simulink model "LastModelb4gameday"  (R2022b)
settings: Solver=FixedStepAuto  StartTime=0.0  StopTime=inf  RelTol=1e-3  EnableMultiTasking=on
libraries: vexarmcortexlib x18
settings Model: ExtModeTrigDuration=25  Creator=Mihai Nicoara  LastModifiedBy=bobsi
settings SolverCC: AutoInsertRateTranBlk=on
settings OptimizationCC: EnhancedBackFolding=on  PassReuseOutputArgsAs=Individual arguments  ZeroExternalMemoryAtStartup=off  ZeroInternalMemoryAtStartup=off  MaxStackSize=64  OptimizeBlockOrder=speed  DifferentSizesBufferReuse=on  OptimizationCustomize=off  EfficientTunableParamExpr=on
settings DebuggingCC: ParameterTunabilityLossMsg=error
settings HardwareCC: ProdBitPerPointer=32  ProdBitPerSizeT=32  ProdBitPerPtrDiffT=32  ProdLargestAtomicInteger=Long  ProdLargestAtomicFloat=Double  ProdWordSize=32  ProdHWDeviceType=ARM Compatible->ARM Cortex
settings SFSimCC: MATLABDynamicMemAlloc=off
settings RTWCC: Description=Embedded Coder  SystemTargetFile=ert.tlc  HardwareBoard=ARM Cortex-based VEX Microcontroller  TLCOptions="-aInlineSetEventsForThisBaseRateFcn=TLC_FALSE -aSuppressMultiTaskScheduler=TLC_FALSE  -aRateBasedStepFcn=0"  TemplateMakefile=ert_default_tmf  Toolchain=GNU Tools for VEX ARM Cortex
settings CodeAppCC: ForceParamTrailComments=on  IgnoreCustomStorageClasses=off  OperatorAnnotations=on  SimulinkDataObjDesc=on  SFDataObjDesc=on  InsertBlockDesc=on
settings ERTTargetCC: ExtModeTransport=1  ExtModeMexFile=ext_serial_win32_comm

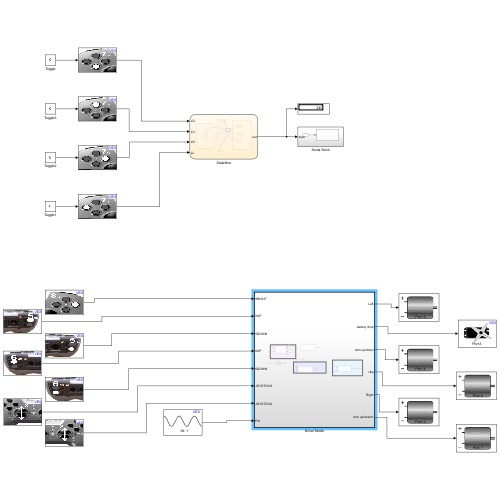
[thumbnail: Simulink's stored preview of the top-level diagram]
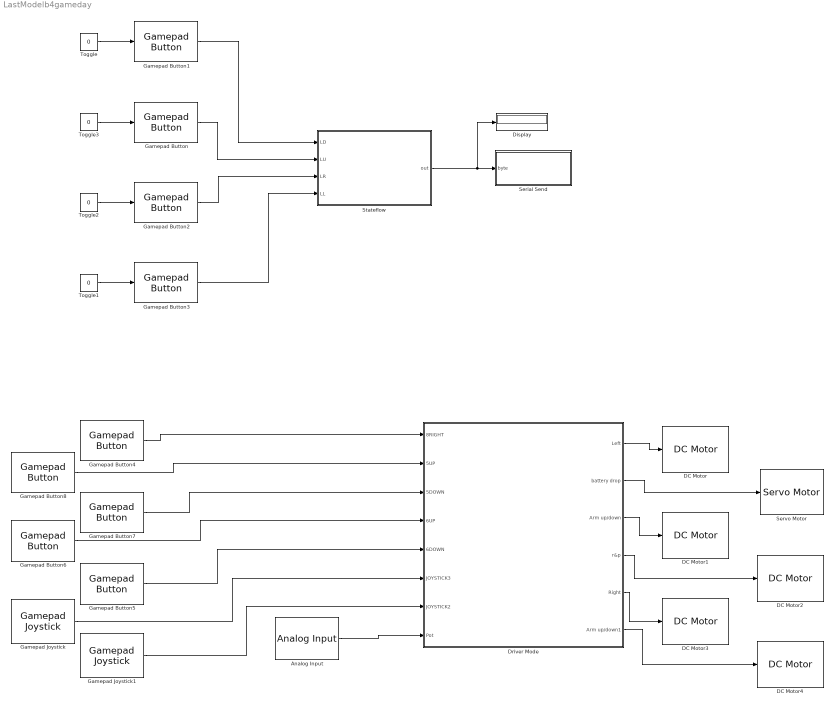
== system LastModelb4gameday ==
  Analog Input : vexarmcortexlib/Sensors/Analog Input  inChan=1  SimulationIn=off  SampleTime=0.02
  DC Motor : vexarmcortexlib/Actuators/DC Motor  motor=9  scaleFactor=1/13.5  SimulationOut=off
  DC Motor1 : vexarmcortexlib/Actuators/DC Motor  motor=4  scaleFactor=1/13.5  SimulationOut=off
  DC Motor2 : vexarmcortexlib/Actuators/DC Motor  motor=6  scaleFactor=1/13.5  SimulationOut=off
  DC Motor3 : vexarmcortexlib/Actuators/DC Motor  motor=2  scaleFactor=1/13.5  SimulationOut=off
  DC Motor4 : vexarmcortexlib/Actuators/DC Motor  motor=7  scaleFactor=1/13.5  SimulationOut=off
  Display : Display
  Driver Mode : Subsystem  TreatAsAtomicUnit=on
  Gamepad Button : vexarmcortexlib/Gamepad/Gamepad Button  joystick=1  chan=7  button56=Up  button78=Up  SimulationIn=on  SampleTime=0.02
  Gamepad Button1 : vexarmcortexlib/Gamepad/Gamepad Button  joystick=1  chan=7  button56=Up  button78=Down  SimulationIn=on  SampleTime=0.02
  Gamepad Button2 : vexarmcortexlib/Gamepad/Gamepad Button  joystick=1  chan=7  button56=Up  button78=Right  SimulationIn=on  SampleTime=0.02
  Gamepad Button3 : vexarmcortexlib/Gamepad/Gamepad Button  joystick=1  chan=7  button56=Up  button78=Left  SimulationIn=on  SampleTime=0.02
  Gamepad Button4 : vexarmcortexlib/Gamepad/Gamepad Button  joystick=1  chan=8  button56=Up  button78=Right  SimulationIn=off  SampleTime=0.02
  Gamepad Button5 : vexarmcortexlib/Gamepad/Gamepad Button  joystick=1  chan=6  button56=Down  button78=Left  SimulationIn=off  SampleTime=0.02
  Gamepad Button6 : vexarmcortexlib/Gamepad/Gamepad Button  joystick=1  chan=6  button56=Up  button78=Left  SimulationIn=off  SampleTime=0.02
  Gamepad Button7 : vexarmcortexlib/Gamepad/Gamepad Button  joystick=1  chan=5  button56=Down  button78=Left  SimulationIn=off  SampleTime=0.02
  Gamepad Button8 : vexarmcortexlib/Gamepad/Gamepad Button  joystick=1  chan=5  button56=Up  button78=Left  SimulationIn=off  SampleTime=0.02
  Gamepad Joystick : vexarmcortexlib/Gamepad/Gamepad Joystick  joystick=1  chan=3  SimulationIn=off  SampleTime=0.02
  Gamepad Joystick1 : vexarmcortexlib/Gamepad/Gamepad Joystick  joystick=1  chan=2  SimulationIn=off  SampleTime=0.02
  Serial Send : Subsystem
  Servo Motor : vexarmcortexlib/Actuators/Servo Motor  motor=3  scaleFactor=60/127  SimulationOut=off
  Stateflow : Stateflow chart  TreatAsAtomicUnit=on
  Toggle{,1..3} (4 alike) : Constant  Value=0
      settings: OpenFcn=|
      | if strcmp('0',get_param(gcb, 'Value'))                        set_param(gcb, 'Value', '1');
      | else
      |             set_param(gcb, 'Value', '0');
      | end
  wires:
  Gamepad Button/1 -> Stateflow/2(LU)
  Stateflow/1(out) -> Display/1, Serial Send/1(byte)
  Gamepad Button2/1 -> Stateflow/3(LR)
  Gamepad Button3/1 -> Stateflow/4(LL)
  Gamepad Button1/1 -> Stateflow/1(LD)
  Toggle/1 -> Gamepad Button1/1
  Toggle3/1 -> Gamepad Button/1
  Toggle2/1 -> Gamepad Button2/1
  Toggle1/1 -> Gamepad Button3/1
  Gamepad Button4/1 -> Driver Mode/1(8RIGHT)
  Gamepad Button8/1 -> Driver Mode/2(5UP)
  Gamepad Button7/1 -> Driver Mode/3(5DOWN)
  Gamepad Button6/1 -> Driver Mode/4(6UP)
  Gamepad Button5/1 -> Driver Mode/5(6DOWN)
  Gamepad Joystick/1 -> Driver Mode/6(JOYSTICK3)
  Gamepad Joystick1/1 -> Driver Mode/7(JOYSTICK2)
  Driver Mode/1(Left) -> DC Motor/1
  Driver Mode/5(Right) -> DC Motor3/1
  Driver Mode/3(Arm up/down) -> DC Motor1/1
  Driver Mode/2(battery drop) -> Servo Motor/1
  Driver Mode/4(r&p) -> DC Motor2/1
  Driver Mode/6(Arm up/down1) -> DC Motor4/1
  Analog Input/1 -> Driver Mode/8(Pot)

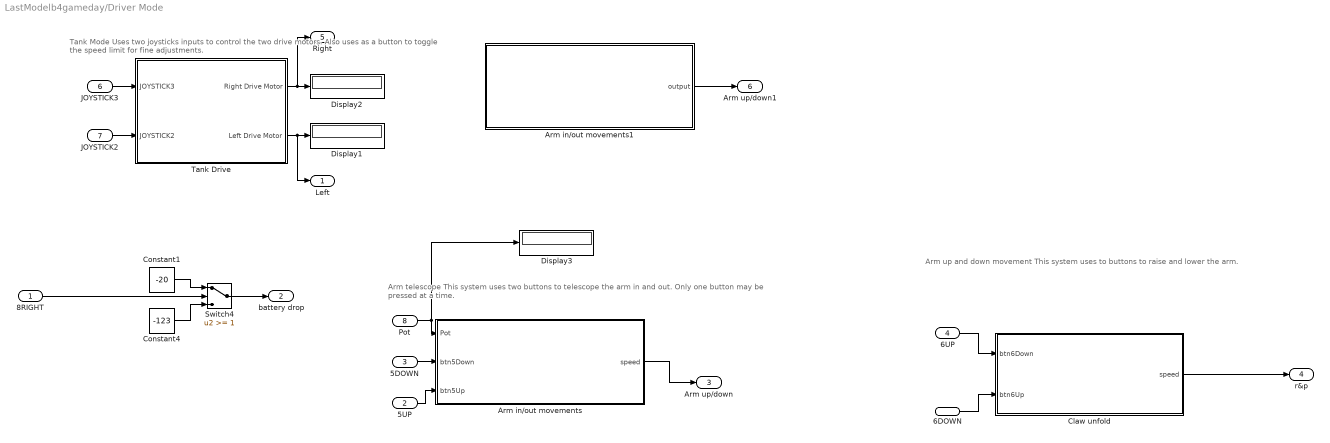
== system LastModelb4gameday/Driver Mode ==
  note: Tank Mode
      | Uses two joysticks inputs to control the two drive motors. Also uses as a button
      | to toggle the speed limit for fine adjustments.
  note: Arm up and down movement
      | This system uses to buttons to raise and lower the arm.
  note: Arm telescope
      | This system uses two buttons to telescope the arm in and out.
      | Only one button may be pressed at a time.
  8RIGHT : Inport
  5UP : Inport  Port=2
  5DOWN : Inport  Port=3
  6UP : Inport  Port=4
  6DOWN : Inport  Port=5
  JOYSTICK3 : Inport  Port=6
  JOYSTICK2 : Inport  Port=7
  Pot : Inport  Port=8
  Arm in/out movements : Stateflow chart  TreatAsAtomicUnit=on
  Arm in/out movements1 : Stateflow chart  TreatAsAtomicUnit=on
  Claw unfold : Stateflow chart  TreatAsAtomicUnit=on
  Constant1 : Constant  Value=-20
  Constant4 : Constant  Value=-123
  Display1 : Display
  Display2 : Display
  Display3 : Display
  Switch4 : Switch  Threshold=1  SaturateOnIntegerOverflow=off  InputSameDT=off
  "Tank Drive " : Subsystem  TreatAsAtomicUnit=on
  Left : Outport
  battery drop : Outport  Port=2
  Arm up/down : Outport  Port=3
  r&p : Outport  Port=4
  Right : Outport  Port=5
  Arm up/down1 : Outport  Port=6
  wires:
  Constant1/1 -> Switch4/1
  Claw unfold/1(speed) -> r&p/1
  Switch4/1 -> battery drop/1
  "Tank Drive "/2(Left Drive Motor) -> Left/1, Display1/1
  "Tank Drive "/1(Right Drive Motor) -> Right/1, Display2/1
  JOYSTICK2/1 -> "Tank Drive "/2(JOYSTICK2)
  8RIGHT/1 -> Switch4/2
  JOYSTICK3/1 -> "Tank Drive "/1(JOYSTICK3)
  Arm in/out movements/1(speed) -> Arm up/down/1
  Constant4/1 -> Switch4/3
  6UP/1 -> Claw unfold/1(btn6Down)
  6DOWN/1 -> Claw unfold/2(btn6Up)
  5UP/1 -> Arm in/out movements/3(btn5Up)
  5DOWN/1 -> Arm in/out movements/2(btn5Down)
  Pot/1 -> Arm in/out movements/1(Pot), Display3/1
  Arm in/out movements1/1(output) -> Arm up/down1/1

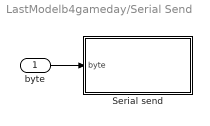
== system LastModelb4gameday/Serial Send ==
  byte : Inport  OutDataTypeStr=uint8  PortDimensions=[1 1]
  Serial send : MATLAB Function  TreatAsAtomicUnit=on
  wires:
  byte/1 -> Serial send/1(byte)

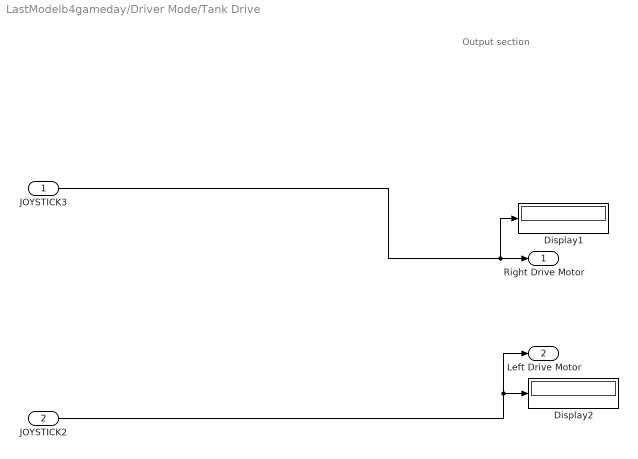
== system LastModelb4gameday/Driver Mode/Tank Drive  ==
  note: Output section
  JOYSTICK3 : Inport
  JOYSTICK2 : Inport  Port=2
  Display1 : Display
  Display2 : Display
  Right Drive Motor : Outport
  Left Drive Motor : Outport  Port=2
  wires:
  JOYSTICK3/1 -> Display1/1, Right Drive Motor/1
  JOYSTICK2/1 -> Display2/1, Left Drive Motor/1

== stateflow chart LastModelb4gameday/Driver Mode/Arm in//out movements1 ==
  state start
    entry:
    output = 1;
  state next
    entry:
    output = 5;
  state after
    entry:
    output = 10;
  state andlast
    entry:
    output = 50;
  state last
    entry:
    output = 100;
  (default) -> start
  last -> start : [after(1,sec)]
  start -> next : [after(1,sec)]
  next -> after : [after(1,sec)]
  after -> andlast : [after(1,sec)]
  andlast -> last : [after(1,sec)]
  data: output output

== matlab function LastModelb4gameday/Serial Send/Serial send ==
  data: byte input
function fcn(byte)
% Serial send single byte
%#codegen

% Config
port = 'uart1';
baud = uint32(600);

persistent isFirstRun

if coder.target('Rtw')
    coder.cinclude('API.h');
    coder.cinclude('string.h');
    file = coder.opaque('FILE *', port,'HeaderFile','API.h');

    if isempty(isFirstRun)
        % first time setup
        isFirstRun = false;

        flags = coder.opaque('uint16', 'SERIAL_8N1');
        coder.ceval('usartInit', file, baud, flags);
    end

    coder.ceval('fputc', byte, file);

end

end

== stateflow chart LastModelb4gameday/Driver Mode/Arm in//out movements ==
  state Recover1
    entry:
    speed = 20
  state ARMDOWN
    entry:
    speed = -80;
  state STOPPED
    entry:
    speed = 0;
  state ARMUP
    entry:
    speed = 80;
  state Recover
    entry:
    speed = 20
  Recover1 -> ARMUP [order 2] : [btn5Down == 0 && btn5Up == 1 ]
  Recover1 -> ARMDOWN [order 3] : [btn5Down == 1 && btn5Up == 0]
  ARMUP -> Recover1 [order 4] : [Pot >= 3080 && btn5Down == 0 && btn5Up == 0]
  ARMDOWN -> Recover1 [order 4] : [Pot >= 3080 && btn5Down == 0 && btn5Up == 0]
  Recover1 -> STOPPED [order 1] : [Pot >= 3080]
  STOPPED -> Recover1 [order 4] : [Pot <= 3080 && btn5Down == 0 && btn5Up == 0]
  (default) -> STOPPED
  STOPPED -> ARMUP [order 1] : [btn5Down == 0 && btn5Up == 1 ]
  STOPPED -> ARMDOWN [order 2] : [btn5Down == 1 && btn5Up == 0]
  ARMDOWN -> STOPPED [order 2] : [btn5Down == 0]
  ARMUP -> STOPPED [order 2] : [btn5Up == 0]
  Recover -> ARMDOWN [order 3] : [btn5Down == 1 && btn5Up == 0]
  ARMDOWN -> Recover [order 3] : [Pot >= 2700 && btn5Down == 0 && btn5Up == 0]
  ARMDOWN -> STOPPED [order 1] : [btn5Down == 1 && btn5Up == 1]
  STOPPED -> Recover [order 3] : [Pot <= 2700 && btn5Down == 0 && btn5Up == 0]
  ARMUP -> STOPPED [order 1] : [btn5Down == 1 && btn5Up == 1]
  Recover -> STOPPED [order 1] : [Pot >= 2900 ]
  ARMUP -> Recover [order 3] : [Pot >= 2700 && btn5Down == 0 && btn5Up == 0]
  Recover -> ARMUP [order 2] : [btn5Down == 0 && btn5Up == 1 ]
  data: Pot input; btn5Down input; btn5Up input; speed output

== stateflow chart LastModelb4gameday/Driver Mode/Claw unfold ==
  state ARMDOWN
    entry:
    speed = -140;
  state STOPPED
    entry:
    speed = 0;
  state ARMUP
    entry:
    speed = 140;
  (default) -> STOPPED
  STOPPED -> ARMUP [order 1] : [btn6Down == 0 && btn6Up == 1 ]
  STOPPED -> ARMDOWN [order 2] : [btn6Down == 1 && btn6Up == 0]
  ARMDOWN -> STOPPED [order 2] : [btn6Down == 0]
  ARMUP -> STOPPED [order 2] : [btn6Up == 0]
  ARMDOWN -> STOPPED [order 1] : [btn6Down == 1 && btn6Up == 1]
  ARMUP -> STOPPED [order 1] : [btn6Down == 1 && btn6Up == 1]
  data: speed output; btn6Down input; btn6Up input

== stateflow chart LastModelb4gameday/Stateflow ==
  state Speed Adjustments [group]
    state speedHigh
      entry:
      out = 0xC3;
  state Squeaky Movements [group]
    state LiftMid
      entry:
      out = 0x5A;
    state driveMid
      entry:
      out = 0x33;
    state rotateMid
      entry:
      out = 0x66;
  state Rotational Adjustments [group]
    state rotLow
      entry:
      out = 0x69;
    state RotHigh
      entry:
      out = 0x0F;
  state Default_Flash
    entry:
    out = 0xF0;
  state MasterFeildReset
    entry:
    out = 0xAA;
  Default_Flash -> speedHigh [order 4] : [LL == 1 && LU == 1]
  speedHigh -> Default_Flash : [after(0.5,sec)]
  Default_Flash -> LiftMid [order 1] : [LL == 1]
  LiftMid -> Default_Flash : [after(0.5,sec)]
  (default) -> Default_Flash
  Default_Flash -> rotLow [order 5] : [LL == 1 && LR == 1]
  rotLow -> Default_Flash : [after(0.5,sec)]
  Default_Flash -> RotHigh [order 6] : [LU == 1 && LD == 1]
  RotHigh -> Default_Flash : [after(0.5,sec)]
  Default_Flash -> MasterFeildReset [order 7] : [LU == 1 && LD == 1 && LR == 1 && LL == 1]
  MasterFeildReset -> Default_Flash : [after(0.5,sec)]
  rotateMid -> Default_Flash : [after(0.5,sec)]
  Default_Flash -> driveMid [order 3] : [LR == 1]
  driveMid -> Default_Flash : [after(0.5,sec)]
  Default_Flash -> rotateMid [order 2] : [LD == 1]
  data: LD input; LU input; out output; LR input; LL input
